simulink model "vehiclefollowing"  (R2022b)
settings: Solver=VariableStepAuto  StartTime=0.0  StopTime=50  RelTol=1e-3
libraries: sim3dautolib x4, simulink x3, vrlib x2, mpcadaslib x2, sim3dlib x1, robotmobilelib x1, slpidlib x1
settings Model: Creator=siva  LastModifiedBy=siva

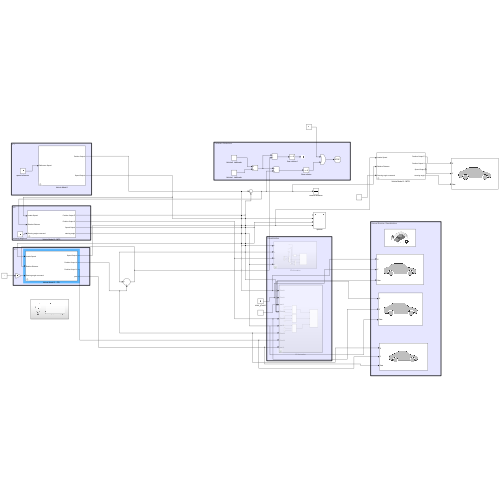
[thumbnail: Simulink's stored preview of the top-level diagram]
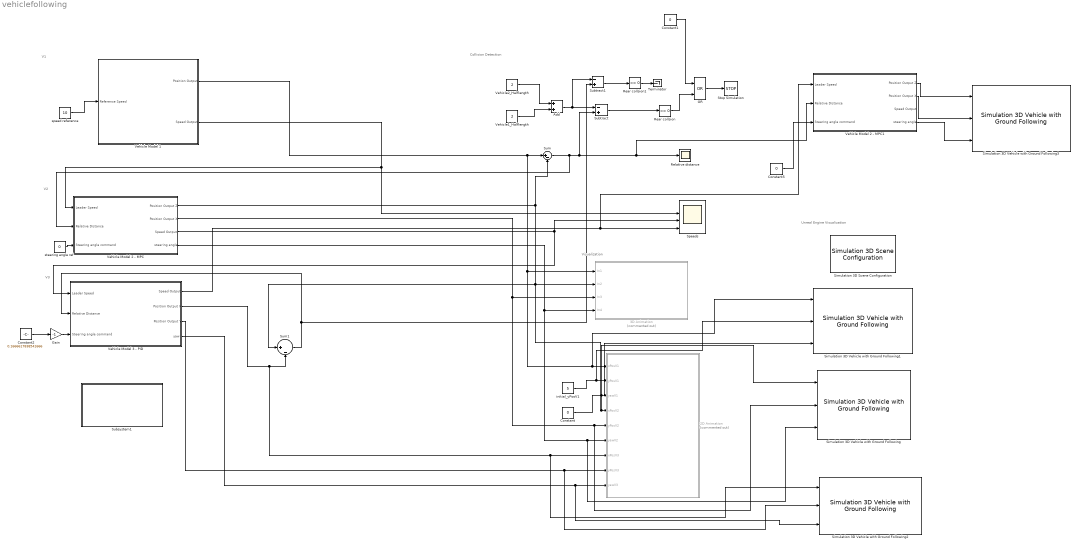
== system vehiclefollowing ==
  note: Unreal Engine Visualization
  note: V3
  note: V2
  note: V1
  note: Visualization
  note: Collision Detection
  2D Animation : Subsystem  Commented=on  TreatAsAtomicUnit=on  SystemSampleTime=0.02
  3D Animation : Subsystem  Commented=on
  Add : Sum
  Constant : Constant  Value=0
  Constant1 : Constant  Value=0
  Constant2 : Constant  Value=0.1666617838541666
  Constant5 : Constant  Value=0
  Gain : Gain  Gain=-1
  OR : Logic  Operator=OR  IconShape=distinctive  AllPortsSameDT=off  OutDataTypeStr=boolean
  Rear collsion : simulink/Logic and Bit Operations/Compare To Constant  relop=<=  const=0  OutDataTypeStr=boolean
  Rear collsion1 : simulink/Logic and Bit Operations/Compare To Constant  relop=<=  const=0  OutDataTypeStr=boolean
  Relative distance : Scope
  Simulation 3D Scene Configuration : sim3dlib/Simulation 3D Scene Configuration  Priority=0  ProjectFormat=Default Scenes  SceneDesc=Straight road  ProjectName=C:\Program Files\MATLAB\R2022b\toolbox\shared\sim3d_projects\automotive_project\UE4\WindowsNoEditor\VehicleSimulation.exe  ScenePath=/Game/Maps/HwStrght  EnableOpenDRIVE=off  vehTagList={'Scene Origin';'SimulinkVehicle1';'SimulinkVehicle2';'SimulinkVehicle3';'SimulinkVehicle4'}  vehTag=SimulinkVehicle3  OpVisEn=off  Ts=0.1  EnableWindow=on  EnableRemoteAccess=off  EnableWeather=off  SunAltitude=40.0  SunAzimuth=90  clouds=10  wind=1  fog=0  rain=0  EnableGeospatial=off  OriginHeight=200  OriginLatitude=40.744652  OriginLongitude=-73.988864  MapStyle=Aerial  AdditionalAssetIDs=[]  UseAdvancedSunSky=off  SolarTime=11  TimeZone=-5  Day=21  Month=9  Year=2022  UseDaylightSavingTime=on  DSTStartDay=10  DSTStartMonth=3  DSTEndDay=3  DSTEndMonth=11  DSTSwitchHour=2  sensorTag=MainCamera1  sensorId=1  sensorName=MainCamera1  mountLoc=Origin  offsetFlag=off  tmountOffset=[0, 0, 0]  rmountOffset=[0, 0, 0]  HorizontalResolution=1280  VerticalResolution=720  HorizontalFOV=60  mountPoint=[0 0 0]  mountOrientation=[0 0 0]  aMode=3  ID=1  GeoTrigger=Inactive
      settings: LibrarySourceBlock=drivingsim3d/Simulation 3D Scene Configuration
  Simulation 3D Vehicle with Ground Following : sim3dautolib/Simulation 3D Vehicle with Ground Following  Priority=-1  PassVehMesh=Hatchback  MeshPath=/MathWorksAutomotiveContent/Vehicles/Muscle/Meshes/SK_MuscleCar.SK_MuscleCar  TrackWidth=1.9  WheelBase=3  WheelRadius=0.35  VehColor=Red  InitialPos=[20, 0, 0]  InitialRot=[0, 0, 0]  ActorName=SimulinkVehicle2  SampleTime=0.1  ActorType=SimulinkVehicle  ID=2  aMode=3  ActorTag=SimulinkVehicle2  CoordinateScheme=ISO  VehLightsControl=off  HeadlightColor=[ 1, 1, 1 ]  HighBeamIntensity=100000  LowBeamIntensity=60000  HighBeamConeAngle=70  LowBeamConeAngle=70  LeftHeadlightOrientation=[ 0, 0 ]  RightHeadlightOrientation=[ 0, 0 ]  BrakelightIntensity=500  ReverselightIntensity=500  SignallightIntensity=500  SignallightPeriod=1  SignalPulseWidth=50  TransformOutportEnabled=off
      settings: LibrarySourceBlock=drivingsim3d/Simulation 3D Vehicle with Ground Following
  Simulation 3D Vehicle with Ground Following1 : sim3dautolib/Simulation 3D Vehicle with Ground Following  Priority=-1  PassVehMesh=Small pickup truck  MeshPath=/MathWorksAutomotiveContent/Vehicles/Muscle/Meshes/SK_MuscleCar.SK_MuscleCar  TrackWidth=1.9  WheelBase=3  WheelRadius=0.35  VehColor=Orange  InitialPos=[40, 0, 0]  InitialRot=[0, 0, 0]  ActorName=SimulinkVehicle1  SampleTime=0.1  ActorType=SimulinkVehicle  ID=1  aMode=3  ActorTag=SimulinkVehicle1  CoordinateScheme=ISO  VehLightsControl=off  HeadlightColor=[ 1, 1, 1 ]  HighBeamIntensity=100000  LowBeamIntensity=60000  HighBeamConeAngle=70  LowBeamConeAngle=70  LeftHeadlightOrientation=[ 0, 0 ]  RightHeadlightOrientation=[ 0, 0 ]  BrakelightIntensity=500  ReverselightIntensity=500  SignallightIntensity=500  SignallightPeriod=1  SignalPulseWidth=50  TransformOutportEnabled=off
      settings: LibrarySourceBlock=drivingsim3d/Simulation 3D Vehicle with Ground Following
  Simulation 3D Vehicle with Ground Following2 : sim3dautolib/Simulation 3D Vehicle with Ground Following  Priority=-1  PassVehMesh=Sedan  MeshPath=/MathWorksAutomotiveContent/Vehicles/Muscle/Meshes/SK_MuscleCar.SK_MuscleCar  TrackWidth=1.9  WheelBase=3  WheelRadius=0.35  VehColor=Silver  InitialPos=[0, 0, 0]  InitialRot=[0, 0, 0]  ActorName=SimulinkVehicle3  SampleTime=0.1  ActorType=SimulinkVehicle  ID=3  aMode=3  ActorTag=SimulinkVehicle3  CoordinateScheme=ISO  VehLightsControl=off  HeadlightColor=[ 1, 1, 1 ]  HighBeamIntensity=100000  LowBeamIntensity=60000  HighBeamConeAngle=70  LowBeamConeAngle=70  LeftHeadlightOrientation=[ 0, 0 ]  RightHeadlightOrientation=[ 0, 0 ]  BrakelightIntensity=500  ReverselightIntensity=500  SignallightIntensity=500  SignallightPeriod=1  SignalPulseWidth=50  TransformOutportEnabled=off
      settings: LibrarySourceBlock=drivingsim3d/Simulation 3D Vehicle with Ground Following
  Simulation 3D Vehicle with Ground Following3 : sim3dautolib/Simulation 3D Vehicle with Ground Following  Priority=-1  PassVehMesh=Small pickup truck  MeshPath=/MathWorksAutomotiveContent/Vehicles/Muscle/Meshes/SK_MuscleCar.SK_MuscleCar  TrackWidth=1.9  WheelBase=3  WheelRadius=0.35  VehColor=Black  InitialPos=[80,0, 0]  InitialRot=[0, 0, 0]  ActorName=SimulinkVehicle4  SampleTime=0.1  ActorType=SimulinkVehicle  ID=4  aMode=3  ActorTag=SimulinkVehicle4  CoordinateScheme=ISO  VehLightsControl=off  HeadlightColor=[ 1, 1, 1 ]  HighBeamIntensity=100000  LowBeamIntensity=60000  HighBeamConeAngle=70  LowBeamConeAngle=70  LeftHeadlightOrientation=[ 0, 0 ]  RightHeadlightOrientation=[ 0, 0 ]  BrakelightIntensity=500  ReverselightIntensity=500  SignallightIntensity=500  SignallightPeriod=1  SignalPulseWidth=50  TransformOutportEnabled=off
      settings: LibrarySourceBlock=drivingsim3d/Simulation 3D Vehicle with Ground Following
  Speeds : Scope  NumInputPorts=4
  Stop Simulation : Stop
  Subsystem1 : Subsystem
  Subtract : Sum  Inputs=-+
  Subtract1 : Sum  Inputs=-+
  Sum : Sum  Inputs=|+-
  Sum1 : Sum  Inputs=|+-
  Terminator : Terminator
  Vehicle Model 1 : Subsystem  mask{Pos=40, Speed=20}
      mask prompts: Pos "Initial Position"; Speed "Initial Speed"
      mask TypeOptions Pos: Initial Position/Value
      mask TypeOptions Speed: Initial Speed/Value
  Vehicle Model 2 - MPC : Subsystem  mask{Pos=20, Speed=25}
      mask prompts: Pos "Initial Position"; Speed "Initial Speed"
      mask TypeOptions Pos: Initial Position/Value
      mask TypeOptions Speed: Initial Speed/Value
  Vehicle Model 2 - MPC1 : Subsystem  mask{Pos=80, Speed=20}
      mask prompts: Pos "Initial Position"; Speed "Initial Speed"
      mask TypeOptions Pos: Initial Position/Value
      mask TypeOptions Speed: Initial Speed/Value
  "Vehicle Model 3 - PID " : Subsystem  mask{Pos=0, Speed=20}
      mask prompts: Pos "Initial Position"; Speed "Initial Speed"
      mask TypeOptions Pos: Initial Position X/Value
      mask TypeOptions Speed: Initial Speed/Value
  Vehicle1_Halflength : Constant  Value=2
  Vehicle2_Halflength : Constant  Value=2
  initial_yPosV1 : Constant  Value=5
  speed reference : Constant  Value=10
  steering angle ref : Constant  Value=0
  wires:
  speed reference/1 -> Vehicle Model 1/1(Reference Speed)
  Vehicle Model 1/2(Speed Output) -> Vehicle Model 2 - MPC/1(Leader Speed), Speeds/2
  Vehicle Model 2 - MPC/1(Position Output Z) -> Sum/2, Simulation 3D Vehicle with Ground Following/1, 2D Animation/4(xPosV2), Sum1/1, 3D Animation/2(In2)
  Vehicle Model 2 - MPC/3(Speed Output) -> "Vehicle Model 3 - PID "/1(Leader Speed), Speeds/3
  Sum/1 -> Vehicle Model 2 - MPC/2(Relative Distance), Subtract/2, Vehicle Model 2 - MPC1/2(Relative Distance), Relative distance/1
  steering angle ref/1 -> Vehicle Model 2 - MPC/3(Steering angle command)
  Vehicle Model 2 - MPC/2(Position Output X) -> Simulation 3D Vehicle with Ground Following/2, 2D Animation/5(yPosV2), 3D Animation/3(In3)
  Vehicle Model 2 - MPC/4(steering angle) -> Simulation 3D Vehicle with Ground Following/3, 2D Animation/6(yawV2), 3D Animation/4(In4)
  Vehicle Model 1/1(Position Output) -> Simulation 3D Vehicle with Ground Following1/1, 2D Animation/1(xPosV1), 3D Animation/1(In1), Sum/1
  initial_yPosV1/1 -> Simulation 3D Vehicle with Ground Following1/2, 2D Animation/2(yPosV1)
  Constant/1 -> Simulation 3D Vehicle with Ground Following1/3, 2D Animation/3(yawV1)
  Vehicle2_Halflength/1 -> Add/1
  Vehicle1_Halflength/1 -> Add/2
  Add/1 -> Subtract1/1, Subtract/1
  Subtract/1 -> Rear collsion/1
  "Vehicle Model 3 - PID "/3(Position Output Y) -> Simulation 3D Vehicle with Ground Following2/2, 2D Animation/8(yPosV3)
  "Vehicle Model 3 - PID "/4(yaw) -> Simulation 3D Vehicle with Ground Following2/3, 2D Animation/9(yawV3)
  Constant2/1 -> Gain/1
  Sum1/1 -> "Vehicle Model 3 - PID "/2(Relative Distance), Subtract1/2
  "Vehicle Model 3 - PID "/1(Speed Output) -> Vehicle Model 2 - MPC1/1(Leader Speed), Speeds/4
  Rear collsion/1 -> OR/2
  OR/1 -> Stop Simulation/1
  Subtract1/1 -> Rear collsion1/1
  Constant1/1 -> OR/1
  Rear collsion1/1 -> Terminator/1
  Gain/1 -> "Vehicle Model 3 - PID "/3(Steering angle command)
  "Vehicle Model 3 - PID "/2(Position Output X) -> Simulation 3D Vehicle with Ground Following2/1, 2D Animation/7(xPosV3), Sum1/2
  Vehicle Model 2 - MPC1/1(Position Output Z) -> Simulation 3D Vehicle with Ground Following3/1
  Vehicle Model 2 - MPC1/2(Position Output X) -> Simulation 3D Vehicle with Ground Following3/2
  Vehicle Model 2 - MPC1/4(steering angle) -> Simulation 3D Vehicle with Ground Following3/3
  Constant5/1 -> Vehicle Model 2 - MPC1/3(Steering angle command)

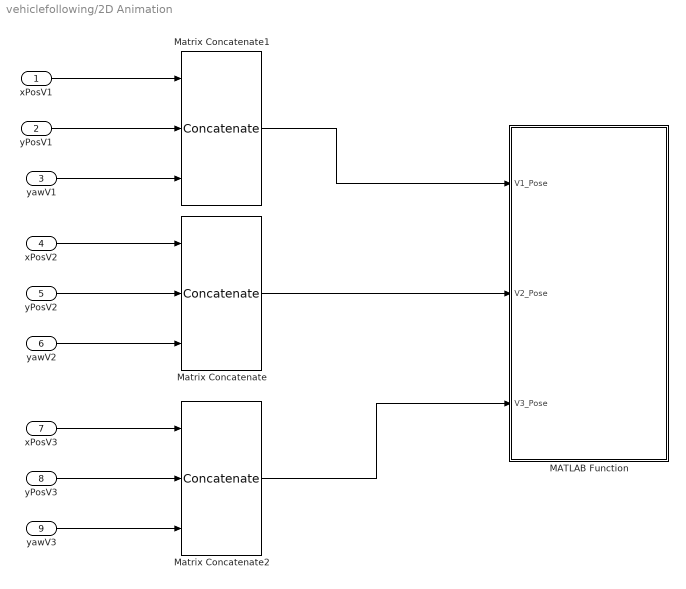
== system vehiclefollowing/2D Animation ==
  xPosV1 : Inport
  yPosV1 : Inport  Port=2
  yawV1 : Inport  Port=3
  xPosV2 : Inport  Port=4
  yPosV2 : Inport  Port=5
  yawV2 : Inport  Port=6
  xPosV3 : Inport  Port=7
  yPosV3 : Inport  Port=8
  yawV3 : Inport  Port=9
  MATLAB Function : MATLAB Function  TreatAsAtomicUnit=on
      mask init:
      | close all;
      | figure('units','normalized','outerPosition',[0 0 1 1]);
      | grid on
      | axis equal
      | hold on
  Matrix Concatenate : Concatenate  NumInputs=3  ConcatenateDimension=2
  Matrix Concatenate1 : Concatenate  NumInputs=3  ConcatenateDimension=2
  Matrix Concatenate2 : Concatenate  NumInputs=3  ConcatenateDimension=2
  wires:
  xPosV2/1 -> Matrix Concatenate/1
  yPosV2/1 -> Matrix Concatenate/2
  yawV2/1 -> Matrix Concatenate/3
  Matrix Concatenate/1 -> MATLAB Function/2(V2_Pose)
  Matrix Concatenate1/1 -> MATLAB Function/1(V1_Pose)
  xPosV1/1 -> Matrix Concatenate1/1
  yawV1/1 -> Matrix Concatenate1/3
  yPosV1/1 -> Matrix Concatenate1/2
  xPosV3/1 -> Matrix Concatenate2/1
  yawV3/1 -> Matrix Concatenate2/3
  yPosV3/1 -> Matrix Concatenate2/2
  Matrix Concatenate2/1 -> MATLAB Function/3(V3_Pose)

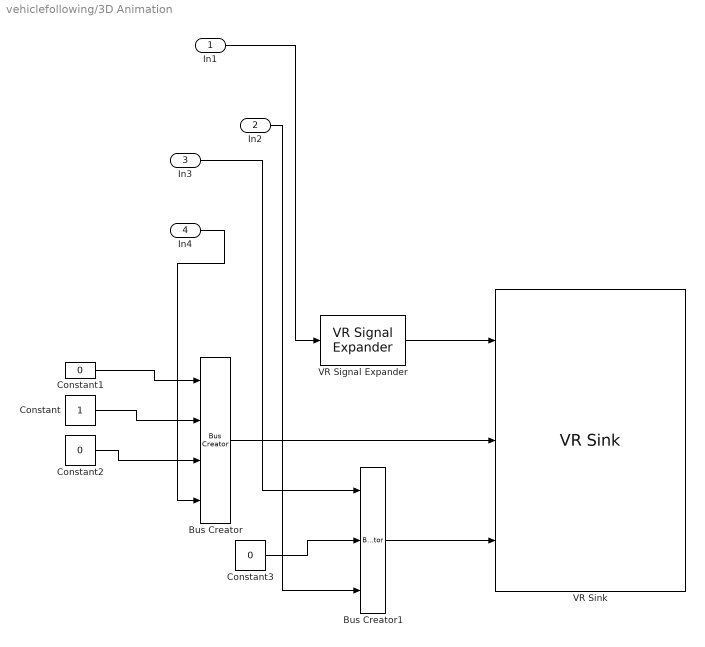
== system vehiclefollowing/3D Animation ==
  In1 : Inport
  In2 : Inport  Port=2
  In3 : Inport  Port=3
  In4 : Inport  Port=4
  Bus Creator : BusCreator  Inputs=4
  Bus Creator1 : BusCreator  Inputs=3
  Constant : Constant
  Constant1 : Constant  Value=0
  Constant2 : Constant  Value=0
  Constant3 : Constant  Value=0
  VR Signal Expander : vrlib/VR Signal Expander  outwidth=3  outidx=[3]
  VR Sink : vrlib/VR Sink  InstantiateOnLoad=on  SampleTime=0.02  ViewEnable=on  RemoteChange=off  RemoteView=off  FieldsWritten=Car_Red.translation.3.1.1.double#Car_Blue.rotation.4.1.1.double#Car_Blue.translation.3.1.1.double  WorldFileName=E:\fyp\PlatoonWorld.WRL  AutoView=off  VideoDimensions=[]  AllowVariableSize=off
  wires:
  Constant1/1 -> Bus Creator/1
  In2/1 -> Bus Creator1/3
  Bus Creator/1 -> VR Sink/2
  Constant3/1 -> Bus Creator1/2
  Bus Creator1/1 -> VR Sink/3
  Constant2/1 -> Bus Creator/3
  VR Signal Expander/1 -> VR Sink/1
  Constant/1 -> Bus Creator/2
  In1/1 -> VR Signal Expander/1
  In4/1 -> Bus Creator/4
  In3/1 -> Bus Creator1/1

== system vehiclefollowing/Subsystem1 ==
  Dashboard Scope : DashboardScope
  Gauge : CircularGaugeBlock
  Knob : KnobBlock  ScaleMin=-0.2  ScaleMax=0.2

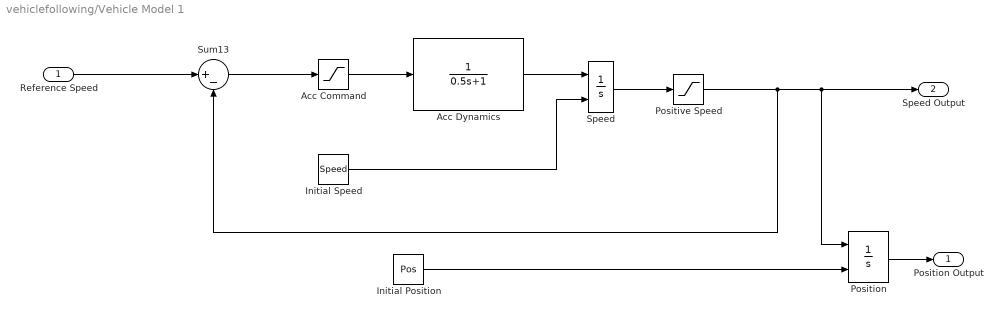
== system vehiclefollowing/Vehicle Model 1 ==
  Reference Speed : Inport
  Acc Command : Saturate  UpperLimit=2  LowerLimit=-3
  Acc Dynamics : TransferFcn  Denominator=[0.5 1]
  Initial Position : Constant  Value=Pos
  Initial Speed : Constant  Value=Speed
  Position : Integrator  InitialConditionSource=external
  Positive Speed : Saturate  UpperLimit=inf  LowerLimit=0
  Speed : Integrator  InitialConditionSource=external
  Sum13 : Sum  Inputs=|+-
  Position Output : Outport  VectorParamsAs1DForOutWhenUnconnected=off
  Speed Output : Outport  Port=2  VectorParamsAs1DForOutWhenUnconnected=off
  wires:
  Speed/1 -> Positive Speed/1
  Positive Speed/1 -> Sum13/2, Speed Output/1, Position/1
  Initial Position/1 -> Position/2
  Sum13/1 -> Acc Command/1
  Reference Speed/1 -> Sum13/1
  Acc Command/1 -> Acc Dynamics/1
  Acc Dynamics/1 -> Speed/1
  Initial Speed/1 -> Speed/2
  Position/1 -> Position Output/1

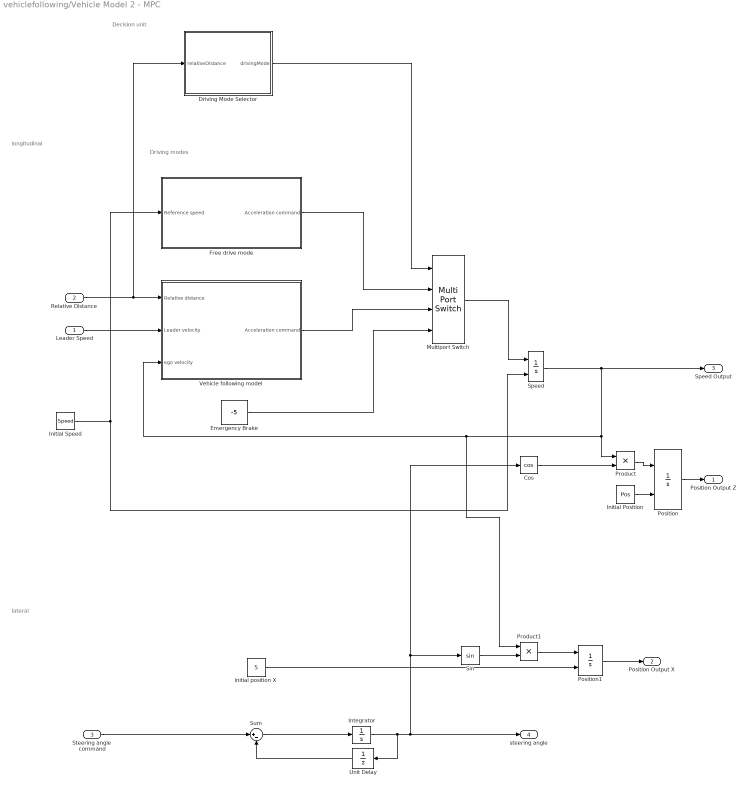
== system vehiclefollowing/Vehicle Model 2 - MPC ==
  note: longitudinal
  note: lateral
  note: Driving modes
  note: Decision unit
  Leader Speed : Inport
  Relative Distance : Inport  Port=2
  Steering angle command : Inport  Port=3
  Cos : Trigonometry  Operator=cos
  Driving Mode Selector : Stateflow chart  TreatAsAtomicUnit=on
  Emergency Brake : Constant  Value=-5
  Free drive mode : Subsystem
  Initial Position : Constant  Value=Pos
  Initial Speed : Constant  Value=Speed
  Integrator : Integrator
  Multiport Switch : MultiPortSwitch  SaturateOnIntegerOverflow=off  InputSameDT=off
  Position : Integrator  InitialConditionSource=external
  Position1 : Integrator  InitialConditionSource=external
  Product : Product
  Product1 : Product
  Sin : Trigonometry
  Speed : Integrator  InitialConditionSource=external  LimitOutput=on  LowerSaturationLimit=0
  Sum : Sum  Inputs=|+-
  Unit Delay : UnitDelay  SampleTime=-1  HasFrameUpgradeWarning=on
  Vehicle following model : Subsystem
  initial position X : Constant  Value=5
  Position Output Z : Outport  VectorParamsAs1DForOutWhenUnconnected=off
  Position Output X : Outport  Port=2  VectorParamsAs1DForOutWhenUnconnected=off
  Speed Output : Outport  Port=3  VectorParamsAs1DForOutWhenUnconnected=off
  steering angle : Outport  Port=4
  wires:
  Driving Mode Selector/1(drivingMode) -> Multiport Switch/1
  Emergency Brake/1 -> Multiport Switch/4
  Multiport Switch/1 -> Speed/1
  Free drive mode/1(Acceleration command) -> Multiport Switch/2
  Vehicle following model/1(Acceleration command) -> Multiport Switch/3
  Leader Speed/1 -> Vehicle following model/2(Leader velocity)
  Relative Distance/1 -> Vehicle following model/1(Relative distance), Driving Mode Selector/1(relativeDistance)
  Position1/1 -> Position Output X/1
  Product1/1 -> Position1/1
  Sin/1 -> Product1/2
  Product/1 -> Position/1
  Cos/1 -> Product/2
  initial position X/1 -> Position1/2
  Unit Delay/1 -> Sum/2
  Integrator/1 -> steering angle/1, Cos/1, Sin/1, Unit Delay/1
  Sum/1 -> Integrator/1
  Steering angle command/1 -> Sum/1
  Position/1 -> Position Output Z/1
  Initial Speed/1 -> Speed/2, Free drive mode/1(Reference speed)
  Initial Position/1 -> Position/2
  Speed/1 -> Product/1, Vehicle following model/3(ego velocity), Product1/1, Speed Output/1

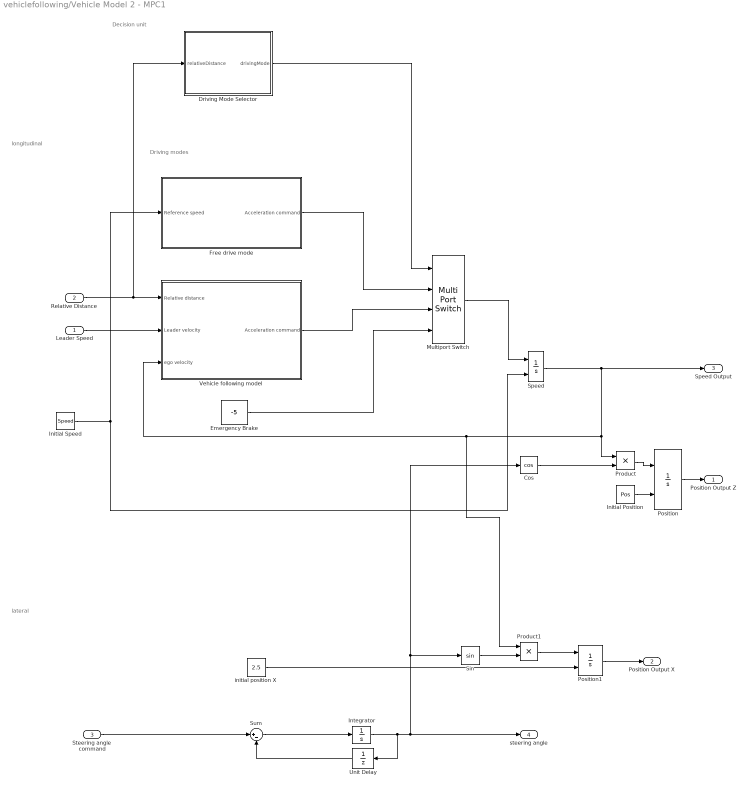
== system vehiclefollowing/Vehicle Model 2 - MPC1 ==
  note: longitudinal
  note: lateral
  note: Driving modes
  note: Decision unit
  Leader Speed : Inport
  Relative Distance : Inport  Port=2
  Steering angle command : Inport  Port=3
  Cos : Trigonometry  Operator=cos
  Driving Mode Selector : Stateflow chart  TreatAsAtomicUnit=on
  Emergency Brake : Constant  Value=-5
  Free drive mode : Subsystem
  Initial Position : Constant  Value=Pos
  Initial Speed : Constant  Value=Speed
  Integrator : Integrator
  Multiport Switch : MultiPortSwitch  SaturateOnIntegerOverflow=off  InputSameDT=off
  Position : Integrator  InitialConditionSource=external
  Position1 : Integrator  InitialConditionSource=external
  Product : Product
  Product1 : Product
  Sin : Trigonometry
  Speed : Integrator  InitialConditionSource=external  LimitOutput=on  LowerSaturationLimit=0
  Sum : Sum  Inputs=|+-
  Unit Delay : UnitDelay  SampleTime=-1  HasFrameUpgradeWarning=on
  Vehicle following model : Subsystem
  initial position X : Constant  Value=2.5
  Position Output Z : Outport  VectorParamsAs1DForOutWhenUnconnected=off
  Position Output X : Outport  Port=2  VectorParamsAs1DForOutWhenUnconnected=off
  Speed Output : Outport  Port=3  VectorParamsAs1DForOutWhenUnconnected=off
  steering angle : Outport  Port=4
  wires:
  Driving Mode Selector/1(drivingMode) -> Multiport Switch/1
  Emergency Brake/1 -> Multiport Switch/4
  Multiport Switch/1 -> Speed/1
  Free drive mode/1(Acceleration command) -> Multiport Switch/2
  Vehicle following model/1(Acceleration command) -> Multiport Switch/3
  Leader Speed/1 -> Vehicle following model/2(Leader velocity)
  Relative Distance/1 -> Vehicle following model/1(Relative distance), Driving Mode Selector/1(relativeDistance)
  Position1/1 -> Position Output X/1
  Product1/1 -> Position1/1
  Sin/1 -> Product1/2
  Product/1 -> Position/1
  Cos/1 -> Product/2
  initial position X/1 -> Position1/2
  Unit Delay/1 -> Sum/2
  Integrator/1 -> steering angle/1, Cos/1, Sin/1, Unit Delay/1
  Sum/1 -> Integrator/1
  Steering angle command/1 -> Sum/1
  Position/1 -> Position Output Z/1
  Initial Speed/1 -> Speed/2, Free drive mode/1(Reference speed)
  Initial Position/1 -> Position/2
  Speed/1 -> Product/1, Vehicle following model/3(ego velocity), Product1/1, Speed Output/1

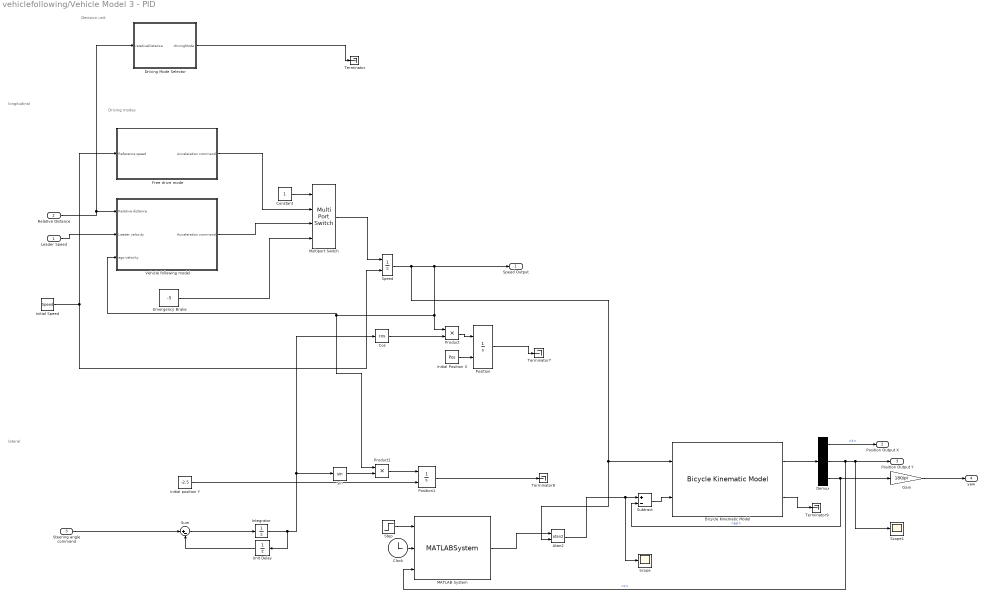
== system vehiclefollowing/Vehicle Model 3 - PID  ==
  note: Decision unit
  note: Driving modes
  note: lateral
  note: longitudinal
  Leader Speed : Inport
  Relative Distance : Inport  Port=2
  Steering angle command : Inport  Port=3
  Atan2 : Trigonometry  Operator=atan2
  Bicycle Kinematic Model : robotmobilelib/Bicycle Kinematic Model  VehicleInputs=Vehicle Speed & Steering Angle  WheelBase=3  VehicleSpeedRange=[0 12]  MaxSteeringAngle=pi/4  InitialState=[0; 5; 0]  SimulateUsing=Interpreted execution
  Clock : Clock
  Constant : Constant
  Cos : Trigonometry  Operator=cos
  Demux : Demux  Outputs=3
  Driving Mode Selector : Stateflow chart  TreatAsAtomicUnit=on
  Emergency Brake : Constant  Value=-5
  Free drive mode : Subsystem
  Gain : Gain  Gain=180/pi
  Initial Position X : Constant  Value=Pos
  Initial Speed : Constant  Value=Speed
  Integrator : Integrator
  MATLAB System : MATLABSystem  System=LaneChanger  SimulateUsing=Interpreted execution
      mask Type: LaneChanger
      mask Display:
      | disp('LaneChanger');
      | port_label('input',1,'flag');
      | port_label('input',2,'clock');
      | port_label('input',3,'y');
      | port_label('output',1,'latSpeed');
  Multiport Switch : MultiPortSwitch  SaturateOnIntegerOverflow=off  InputSameDT=off
  Position : Integrator  InitialConditionSource=external
  Position1 : Integrator  InitialConditionSource=external
  Product : Product
  Product1 : Product
  Scope : Scope
  Scope1 : Scope
  Sin : Trigonometry
  Speed : Integrator  InitialConditionSource=external  LimitOutput=on  UpperSaturationLimit=12  LowerSaturationLimit=0
  Step : Step  Time=3  SampleTime=0
  Subtract : Sum  Inputs=+-
  Sum : Sum  Inputs=|+-
  Terminator{,7..9} (4 alike) : Terminator
  Unit Delay : UnitDelay  SampleTime=-1  HasFrameUpgradeWarning=on
  Vehicle following model : Subsystem
  initial position Y : Constant  Value=-2.5
  Speed Output : Outport  VectorParamsAs1DForOutWhenUnconnected=off
  Position Output X : Outport  Port=2  VectorParamsAs1DForOutWhenUnconnected=off
  Position Output Y : Outport  Port=3  VectorParamsAs1DForOutWhenUnconnected=off
  yaw : Outport  Port=4
  wires:
  Speed/1 -> Atan2/2, Bicycle Kinematic Model/1, Speed Output/1, Product1/1, Vehicle following model/3(ego velocity), Product/1
  Initial Position X/1 -> Position/2
  Initial Speed/1 -> Free drive mode/1(Reference speed), Speed/2
  Position/1 -> Terminator7/1
  Steering angle command/1 -> Sum/1
  Sum/1 -> Integrator/1
  Integrator/1 -> Unit Delay/1, Sin/1, Cos/1
  Unit Delay/1 -> Sum/2
  initial position Y/1 -> Position1/2
  Cos/1 -> Product/2
  Product/1 -> Position/1
  Sin/1 -> Product1/2
  Product1/1 -> Position1/1
  Position1/1 -> Terminator8/1
  Relative Distance/1 -> Driving Mode Selector/1(relativeDistance), Vehicle following model/1(Relative distance)
  Leader Speed/1 -> Vehicle following model/2(Leader velocity)
  Vehicle following model/1(Acceleration command) -> Multiport Switch/3
  Free drive mode/1(Acceleration command) -> Multiport Switch/2
  Multiport Switch/1 -> Speed/1
  Emergency Brake/1 -> Multiport Switch/4
  Driving Mode Selector/1(drivingMode) -> Terminator/1
  Constant/1 -> Multiport Switch/1
  Bicycle Kinematic Model/1 -> Demux/1
  Demux/3 -> Subtract/2, Gain/1  "<psi>"
  Demux/2 -> MATLAB System/3, Scope1/1, Position Output Y/1  "<Y>"
  Demux/1 -> Position Output X/1  "<X>"
  Gain/1 -> yaw/1
  Bicycle Kinematic Model/2 -> Terminator9/1
  Clock/1 -> MATLAB System/2
  Step/1 -> MATLAB System/1
  MATLAB System/1 -> Atan2/1
  Atan2/1 -> Scope/1, Subtract/1
  Subtract/1 -> Bicycle Kinematic Model/2

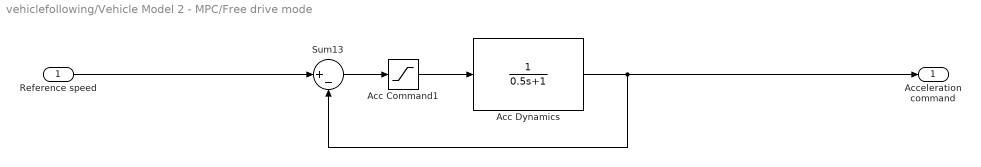
== system vehiclefollowing/Vehicle Model 2 - MPC/Free drive mode ==
  Reference speed : Inport
  Acc Command1 : Saturate  UpperLimit=2  LowerLimit=-3
  Acc Dynamics : TransferFcn  Denominator=[0.5 1]
  Sum13 : Sum  Inputs=|+-
  Acceleration command : Outport
  wires:
  Acc Command1/1 -> Acc Dynamics/1
  Sum13/1 -> Acc Command1/1
  Acc Dynamics/1 -> Acceleration command/1, Sum13/2
  Reference speed/1 -> Sum13/1

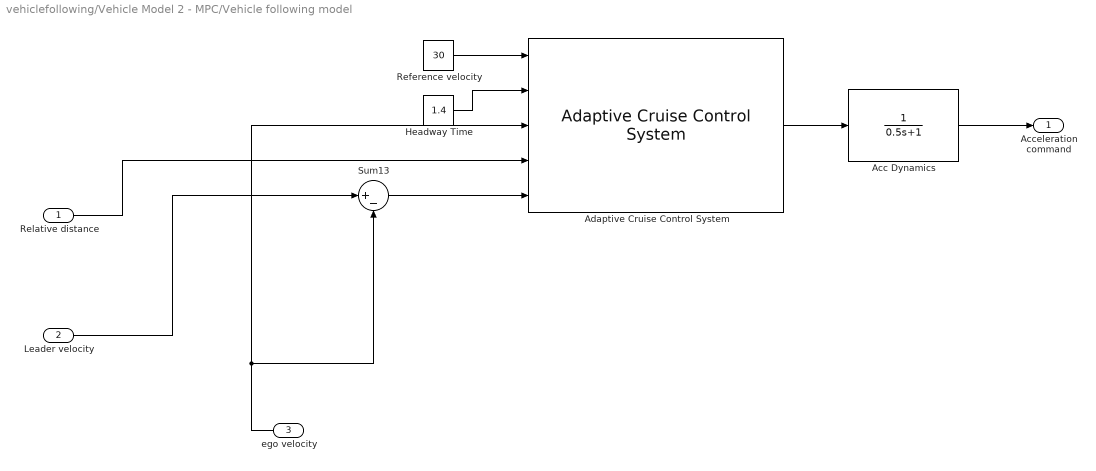
== system vehiclefollowing/Vehicle Model 2 - MPC/Vehicle following model ==
  Relative distance : Inport
  Leader velocity : Inport  Port=2
  ego velocity : Inport  Port=3
  Acc Dynamics : TransferFcn  Denominator=[0.5 1]
  Adaptive Cruise Control System : mpcadaslib/Adaptive Cruise Control System  EgoModel=tf(1,[0.5,1,0])  InitialEgoVelocity=20  DefaultSpacing=10  MaxVelocity=50  MinAcceleration=-3  amin_ext=off  MaxAcceleration=2  amax_ext=off  Ts=0.5  PredictionHorizon=200  ControllerBehavior=0.590  suboptimal=off  maxiter=10  datatypeopt=double  optmode=off  trackmode=off
      settings: LibrarySourceBlock=mpclib/Automated Driving/Adaptive Cruise Control System
  Headway Time : Constant  Value=1.4
  Reference velocity : Constant  Value=30
  Sum13 : Sum  Inputs=|+-
  Acceleration command : Outport
  wires:
  Acc Dynamics/1 -> Acceleration command/1
  Reference velocity/1 -> Adaptive Cruise Control System/1
  Adaptive Cruise Control System/1 -> Acc Dynamics/1
  Leader velocity/1 -> Sum13/1
  Headway Time/1 -> Adaptive Cruise Control System/2
  ego velocity/1 -> Adaptive Cruise Control System/3, Sum13/2
  Sum13/1 -> Adaptive Cruise Control System/5
  Relative distance/1 -> Adaptive Cruise Control System/4

== system vehiclefollowing/Vehicle Model 2 - MPC1/Free drive mode ==
  Reference speed : Inport
  Acc Command1 : Saturate  UpperLimit=2  LowerLimit=-3
  Acc Dynamics : TransferFcn  Denominator=[0.5 1]
  Sum13 : Sum  Inputs=|+-
  Acceleration command : Outport
  wires:
  Acc Command1/1 -> Acc Dynamics/1
  Sum13/1 -> Acc Command1/1
  Acc Dynamics/1 -> Acceleration command/1, Sum13/2
  Reference speed/1 -> Sum13/1

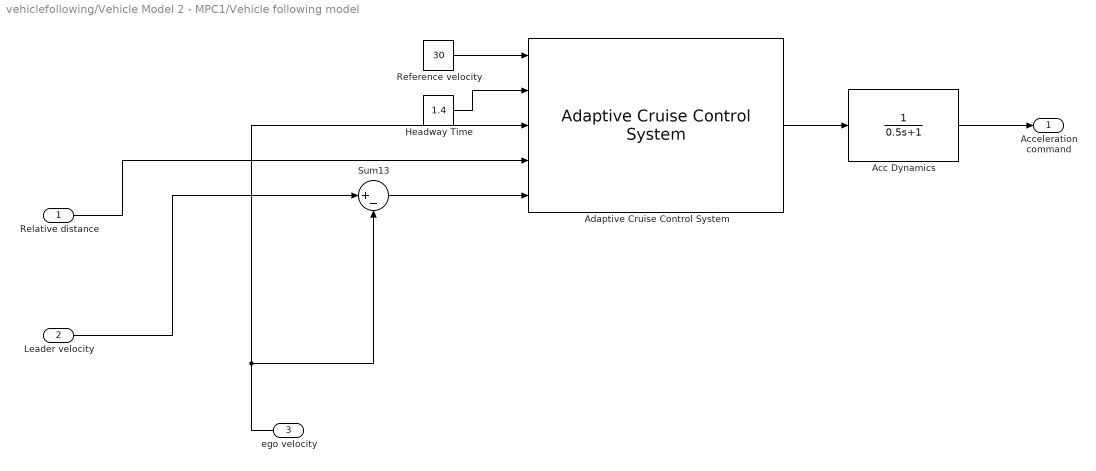
== system vehiclefollowing/Vehicle Model 2 - MPC1/Vehicle following model ==
  Relative distance : Inport
  Leader velocity : Inport  Port=2
  ego velocity : Inport  Port=3
  Acc Dynamics : TransferFcn  Denominator=[0.5 1]
  Adaptive Cruise Control System : mpcadaslib/Adaptive Cruise Control System  EgoModel=tf(1,[0.5,1,0])  InitialEgoVelocity=20  DefaultSpacing=10  MaxVelocity=50  MinAcceleration=-3  amin_ext=off  MaxAcceleration=2  amax_ext=off  Ts=0.5  PredictionHorizon=200  ControllerBehavior=0.590  suboptimal=off  maxiter=10  datatypeopt=double  optmode=off  trackmode=off
      settings: LibrarySourceBlock=mpclib/Automated Driving/Adaptive Cruise Control System
  Headway Time : Constant  Value=1.4
  Reference velocity : Constant  Value=30
  Sum13 : Sum  Inputs=|+-
  Acceleration command : Outport
  wires:
  Acc Dynamics/1 -> Acceleration command/1
  Reference velocity/1 -> Adaptive Cruise Control System/1
  Adaptive Cruise Control System/1 -> Acc Dynamics/1
  Leader velocity/1 -> Sum13/1
  Headway Time/1 -> Adaptive Cruise Control System/2
  ego velocity/1 -> Adaptive Cruise Control System/3, Sum13/2
  Sum13/1 -> Adaptive Cruise Control System/5
  Relative distance/1 -> Adaptive Cruise Control System/4

== system vehiclefollowing/Vehicle Model 3 - PID /Free drive mode ==
  Reference speed : Inport
  Acc Command1 : Saturate  UpperLimit=2  LowerLimit=-3
  Acc Dynamics : TransferFcn  Denominator=[0.5 1]
  Sum13 : Sum  Inputs=|+-
  Acceleration command : Outport
  wires:
  Reference speed/1 -> Sum13/1
  Acc Dynamics/1 -> Sum13/2, Acceleration command/1
  Sum13/1 -> Acc Command1/1
  Acc Command1/1 -> Acc Dynamics/1

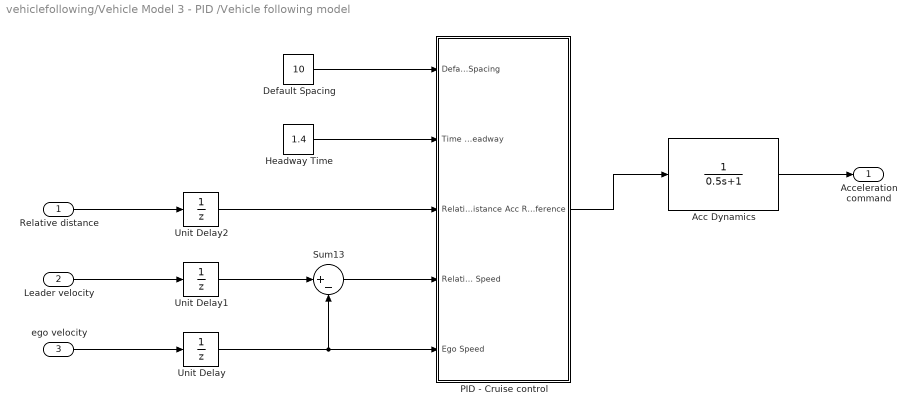
== system vehiclefollowing/Vehicle Model 3 - PID /Vehicle following model ==
  Relative distance : Inport
  Leader velocity : Inport  Port=2
  ego velocity : Inport  Port=3
  Acc Dynamics : TransferFcn  Denominator=[0.5 1]
  Default Spacing : Constant  Value=10
  Headway Time : Constant  Value=1.4
  PID - Cruise control : Subsystem
  Sum13 : Sum  Inputs=|+-
  Unit Delay : UnitDelay  SampleTime=-1  HasFrameUpgradeWarning=on
  Unit Delay1 : UnitDelay  SampleTime=-1  HasFrameUpgradeWarning=on
  Unit Delay2 : UnitDelay  SampleTime=-1  HasFrameUpgradeWarning=on
  Acceleration command : Outport
  wires:
  Relative distance/1 -> Unit Delay2/1
  Sum13/1 -> PID - Cruise control/4(Relative Speed)
  ego velocity/1 -> Unit Delay/1
  Headway Time/1 -> PID - Cruise control/2(Time Headway)
  Leader velocity/1 -> Unit Delay1/1
  PID - Cruise control/1(Acc Reference) -> Acc Dynamics/1
  Default Spacing/1 -> PID - Cruise control/1(Default Spacing)
  Acc Dynamics/1 -> Acceleration command/1
  Unit Delay/1 -> Sum13/2, PID - Cruise control/5(Ego Speed)
  Unit Delay1/1 -> Sum13/1
  Unit Delay2/1 -> PID - Cruise control/3(Relative Distance)

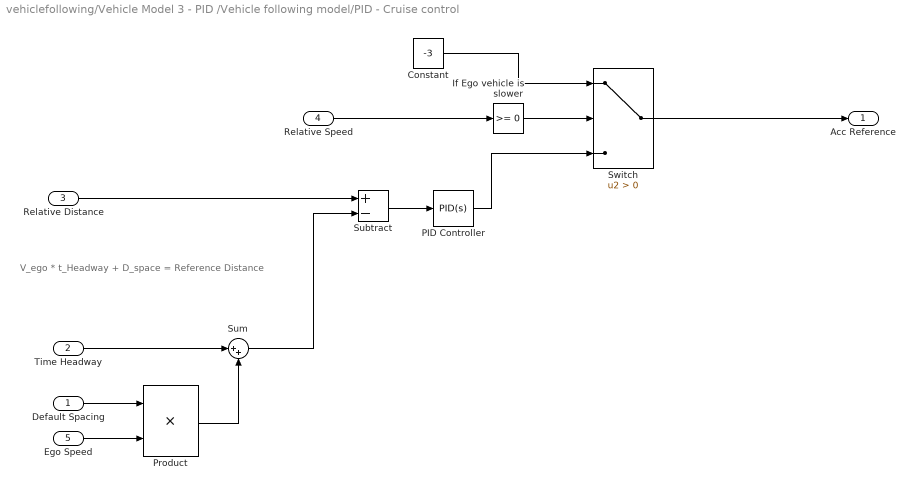
== system vehiclefollowing/Vehicle Model 3 - PID /Vehicle following model/PID - Cruise control ==
  note: V_ego * t_Headway + D_space = Reference Distance
  Default Spacing : Inport
  Time Headway : Inport  Port=2
  Relative Distance : Inport  Port=3
  Relative Speed : Inport  Port=4
  Ego Speed : Inport  Port=5
  Constant : Constant  Value=-3
  If Ego vehicle is slower : simulink/Logic and Bit Operations/Compare To Constant  relop=>=  const=0  OutDataTypeStr=boolean
  PID Controller : slpidlib/PID Controller  Controller=PID  Form=Parallel  TimeDomain=Continuous-time  UseExternalTs=off  SampleTime=-1  IntegratorMethod=Forward Euler  FilterMethod=Forward Euler  ControllerParametersSource=internal  P=2  I=0.04  UseKiTs=off  D=2.1  N=230  UseFilter=on  TunerSelectOption=Transfer Function Based (PID Tuner App)  InitialConditionSource=internal  InitialConditionForIntegrator=0  InitialConditionForFilter=0  DifferentiatorICPrevScaledInput=0  ExternalReset=none  TrackingMode=off  Kt=1  LimitOutput=on  SatLimitsSource=internal  UpperSaturationLimit=2  LowerSaturationLimit=-3  LinearizeAsGain=on  AntiWindupMode=clamping  Kb=1  LimitIntegrator=off  UpperIntegratorSaturationLimit=inf  LowerIntegratorSaturationLimit=-inf  POutMin=[]  POutMax=[]  IOutMin=[]  IOutMax=[]  DOutMin=[]  DOutMax=[]  NOutMin=[]  NOutMax=[]  SumOutMin=[]  SumOutMax=[]  SaturationOutMin=[]  SaturationOutMax=[]  PParamMin=[]  PParamMax=[]  IParamMin=[]  IParamMax=[]  DParamMin=[]  DParamMax=[]  NParamMin=[]  NParamMax=[]  KbParamMin=[]  KbParamMax=[]  KtParamMin=[]  KtParamMax=[]  KbOutMin=[]  KbOutMax=[]  KtOutMin=[]  KtOutMax=[]  IntegratorOutMin=[]  IntegratorOutMax=[]  FilterOutMin=[]  FilterOutMax=[]  SumI1OutMin=[]  SumI1OutMax=[]  SumI2OutMin=[]  SumI2OutMax=[]  SumI3OutMin=[]  SumI3OutMax=[]  SumI4OutMin=[]  SumI4OutMax=[]  SumDOutMin=[]  SumDOutMax=[]  DifferentiatorOutMin=[]  DifferentiatorOutMax=[]  FilterDiffOutCoefMin=[]  FilterDiffOutCoefMax=[]  ReciprocalOutMin=[]  ReciprocalOutMax=[]  SumDenOutMin=[]  SumDenOutMax=[]  SumNumOutMin=[]  SumNumOutMax=[]  DivideOutMin=[]  DivideOutMax=[]  UdiffTsProdOutMin=[]  UdiffTsProdOutMax=[]  NTsProdOutMin=[]  NTsProdOutMax=[]  UintegralTsProdOutMin=[]  UintegralTsProdOutMax=[]  UngainTsProdOutMin=[]  UngainTsProdOutMax=[]  ClampingZeroOutDataTypeStr=Inherit: Inherit via back propagation  ClampingZeroOutMin=[]  ClampingZeroOutMax=[]  FilterDenConstantOutDataTypeStr=Inherit: Inherit via back propagation  FilterDenConstantOutMin=[]  FilterDenConstantOutMax=[]  PCopyOutDataTypeStr=Inherit: Inherit via back propagation  PCopyOutMin=[]  PCopyOutMax=[]  NCopyOutDataTypeStr=Inherit: Inherit via back propagation  NCopyOutMin=[]  NCopyOutMax=[]  IntegratorContinuousStateAttributes=''  IntegratorStateMustResolveToSignalObject=off  IntegratorRTWStateStorageClass=Auto  FilterContinuousStateAttributes=''  FilterStateMustResolveToSignalObject=off  FilterRTWStateStorageClass=Auto  ParallelPVariant=InternalParameters  IdealPVariant=Disabled  IVariant=InternalParameters  DVariant=InternalParameters  IntegratorVariant=Continuous  SatVariant=Enabled  AWVariant=ContClampingParallel  PCopyVariant=Disabled  TRVariant=Disabled  FdbkBlocksVariant=Forward  IdealPFdbkVariant=Disabled  SatFdbkVariant=Disabled  DerivativeFilterVariant=ContFilter  NVariant=InternalParameters  NCopyVariant=Disabled  FilterICVariant=InternalICsFilter  IntegratorICVariant=InternalICs  ExternalResetVariant=Disabled  TRSumVariant=Passthrough  SumFdbkVariant=Disabled  SumVariant=Sum_PID  TsampFilterVariant=InternalTs  TsampNgainVariant=Passthrough  TsampIntegralVariant=Passthrough  ExternalSaturationOutDataTypeStr=Inherit: Same as second input
  Product : Product
  Subtract : Sum  Inputs=+-
  Sum : Sum  Inputs=|++
  Switch : Switch  Criteria=u2 > Threshold  SaturateOnIntegerOverflow=off  InputSameDT=off
  Acc Reference : Outport
  wires:
  Default Spacing/1 -> Product/1
  Ego Speed/1 -> Product/2
  Time Headway/1 -> Sum/1
  Product/1 -> Sum/2
  Relative Distance/1 -> Subtract/1
  Sum/1 -> Subtract/2
  Relative Speed/1 -> If Ego vehicle is slower/1
  If Ego vehicle is slower/1 -> Switch/2
  Subtract/1 -> PID Controller/1
  Switch/1 -> Acc Reference/1
  PID Controller/1 -> Switch/3
  Constant/1 -> Switch/1

== stateflow chart vehiclefollowing/Vehicle Model 2 - MPC/Driving Mode Selector ==
  state FreeDrive
    entry:
    drivingMode = 1;
  state VehicleFollowing
    entry:
    drivingMode = 2;
  state EmergencyBrake
    entry:
    drivingMode =3;
  (default) -> FreeDrive
  VehicleFollowing -> FreeDrive [order 1] : [relativeDistance >50]
  FreeDrive -> VehicleFollowing [order 1] : [relativeDistance <=40]
  FreeDrive -> EmergencyBrake [order 2] : [relativeDistance <=10]
  VehicleFollowing -> EmergencyBrake [order 2] : [relativeDistance <=10]
  EmergencyBrake -> VehicleFollowing : [relativeDistance >15]
  data: relativeDistance input; drivingMode output

== matlab function vehiclefollowing/2D Animation/MATLAB Function ==
  data: V1_Pose input; V2_Pose input; V3_Pose input
function plotVehicle(V1_Pose, V2_Pose, V3_Pose)

%% Clear previous Vehicle
cla;

%% Vehicle 1 - pose

x1 = V1_Pose(1);
y1 = V1_Pose(2);
yaw1 = V1_Pose(3);

centerP = [x1;y1];

V1_HalfLength = 2;
V1_HalfWidth = 1;

% Creating a rectangle
p1= [V1_HalfLength; V1_HalfWidth];
p2= [V1_HalfLength; -V1_HalfWidth];
p3= [-V1_HalfLength; -V1_HalfWidth];
p4= [-V1_HalfLength; V1_HalfWidth];

% Rotation Matrix
Rmatrix = [cos(yaw1) -sin(yaw1); sin(yaw1) cos(yaw1)];

% Rotated points
p1r = centerP + Rmatrix*p1;
p2r = centerP + Rmatrix*p2;
p3r = centerP + Rmatrix*p3;
p4r = centerP + Rmatrix*p4;

% connecting points
Hitbox_V1 = [p1r p2r p3r p4r p1r];

cornersV1_x = transpose(Hitbox_V1(1,:));
cornersV1_y = transpose(Hitbox_V1(2,:));

%% Vehicle 2 - pose

x2 = V2_Pose(1);
y2 = V2_Pose(2);
yaw2 = V2_Pose(3);

centerP = [x2;y2];

V2_HalfLength = 2;
V2_HalfWidth = 1;

% Creating a rectangle
p1= [V2_HalfLength; V2_HalfWidth];
p2= [V2_HalfLength; -V2_HalfWidth];
p3= [-V2_HalfLength; -V2_HalfWidth];
p4= [-V2_HalfLength; V2_HalfWidth];

% Rotation Matrix
Rmatrix = [cos(yaw2) -sin(yaw2); sin(yaw2) cos(yaw2)];

% Rotated points
p1r = centerP + Rmatrix*p1;
p2r = centerP + Rmatrix*p2;
p3r = centerP + Rmatrix*p3;
p4r = centerP + Rmatrix*p4;

% connecting points
Hitbox_V2 = [p1r p2r p3r p4r p1r];

cornersV2_x = transpose(Hitbox_V2(1,:));
cornersV2_y = transpose(Hitbox_V2(2,:));

%% Vehicle 3 - pose

x3 = V3_Pose(1);
y3 = V3_Pose(2);
yaw3 = V3_Pose(3);

centerP = [x3;y3];

V3_HalfLength = 2;
V3_HalfWidth = 1;

% Creating a rectangle
p1= [V3_HalfLength; V3_HalfWidth];
p2= [V3_HalfLength; -V3_HalfWidth];
p3= [-V3_HalfLength; -V3_HalfWidth];
p4= [-V3_HalfLength; V3_HalfWidth];

% Rotation Matrix
Rmatrix = [cos(yaw3) -sin(yaw3); sin(yaw3) cos(yaw3)];

% Rotated points
p1r = centerP + Rmatrix*p1;
p2r = centerP + Rmatrix*p2;
p3r = centerP + Rmatrix*p3;
p4r = centerP + Rmatrix*p4;

% connecting points
Hitbox_V3 = [p1r p2r p3r p4r p1r];

cornersV3_x = transpose(Hitbox_V3(1,:));
cornersV3_y = transpose(Hitbox_V3(2,:));

%% Plot vehicle and the road

plot(cornersV1_x, cornersV1_y,'g'); % Vehicle 1 rectangle
plot(x1,y1,'*'); % Vehicle 1 center

plot(cornersV2_x, cornersV2_y,'r');% vehicle 2 rectangle
plot(x2,y2,'o'); % vehicle 2 center

plot(cornersV3_x, cornersV3_y,'b');% vehicle 3 rectangle
plot(x3,y3,'-'); % vehicle 3 center

upperLine = plot([0,1000], [5,5], 'Color', 'blue');
midLine = plot([0,1000], [0,0], '--', 'Color', 'blue');
lowerLine = plot([0,1000], [-5,-5], 'Color', 'blue');


% Adjust axis
axis([x3-40 x3+40 y3-20 y3+20]);

== stateflow chart vehiclefollowing/Vehicle Model 3 - PID /Driving Mode Selector ==
  state FreeDrive
    entry:
    drivingMode = 1;
  state VehicleFollowing
    entry:
    drivingMode = 2;
  state EmergencyBrake
    entry:
    drivingMode =3;
  (default) -> FreeDrive
  VehicleFollowing -> FreeDrive [order 1] : [relativeDistance >50]
  FreeDrive -> VehicleFollowing [order 1] : [relativeDistance <=0]
  FreeDrive -> EmergencyBrake [order 2] : [relativeDistance <=10]
  VehicleFollowing -> EmergencyBrake [order 2] : [relativeDistance <=10]
  EmergencyBrake -> VehicleFollowing : [relativeDistance >15]
  data: relativeDistance input; drivingMode output

== stateflow chart vehiclefollowing/Vehicle Model 2 - MPC1/Driving Mode Selector ==
  state FreeDrive
    entry:
    drivingMode = 1;
  state VehicleFollowing
    entry:
    drivingMode = 2;
  state EmergencyBrake
    entry:
    drivingMode =3;
  (default) -> FreeDrive
  VehicleFollowing -> FreeDrive [order 1] : [relativeDistance >50]
  FreeDrive -> VehicleFollowing [order 1] : [relativeDistance <=40]
  FreeDrive -> EmergencyBrake [order 2] : [relativeDistance <=10]
  VehicleFollowing -> EmergencyBrake [order 2] : [relativeDistance <=10]
  EmergencyBrake -> VehicleFollowing : [relativeDistance >15]
  data: relativeDistance input; drivingMode output
